simulink subsystem "startOLAE2"  (R2021a)
settings: Solver=VariableStepAuto  StartTime=0.0  StopTime=10.0  RelTol=1e-3
libraries: aerolibutil x3
settings Model: Creator=noraw  LastModifiedBy=noraw

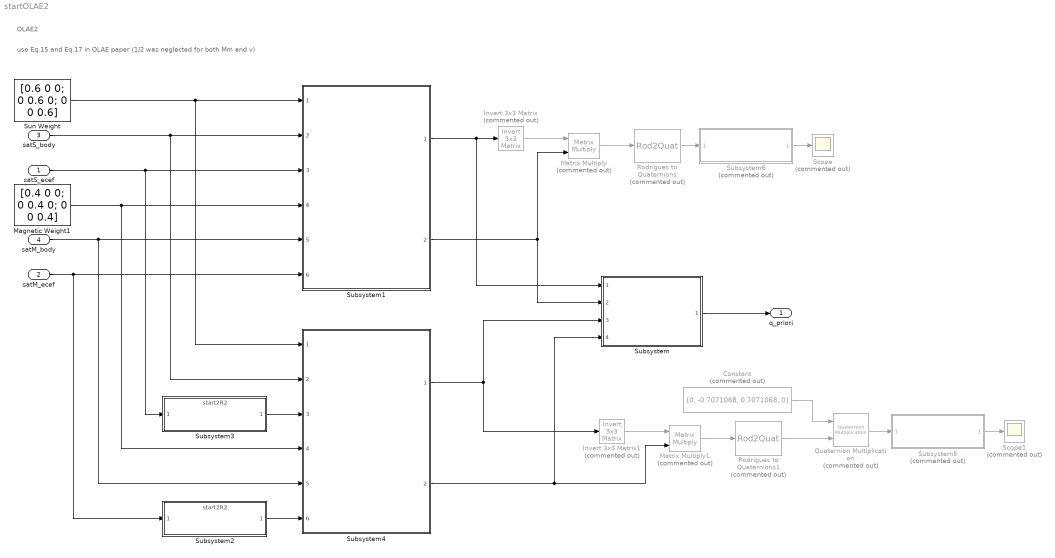
== system startOLAE2 ==
  note: OLAE2
  note: use Eq.15 and Eq.17 in OLAE paper (1/2 was neglected for both Mm and v)
  satS_ecef : Inport  PortDimensions=3
  satM_ecef : Inport  Port=2  PortDimensions=3
  satS_body : Inport  Port=3  PortDimensions=3
  satM_body : Inport  Port=4  PortDimensions=3
  Constant : Constant  Commented=on  Value=[0, -0.7071068, 0.7071068, 0]
  Invert 3x3 Matrix : aerolibutil/Invert  3x3 Matrix  Commented=on
  Invert 3x3 Matrix1 : aerolibutil/Invert  3x3 Matrix  Commented=on
  Magnetic Weight1 : Constant  Value=[0.4 0 0; 0 0.4 0; 0 0 0.4]
  Matrix Multiply : Product  Commented=on  Multiplication=Matrix(*)
  Matrix Multiply1 : Product  Commented=on  Multiplication=Matrix(*)
  Quaternion Multiplication : aerolibutil/Quaternion Multiplication  Commented=on
  Rodrigues to Quaternions : Rod2Quat  Commented=on
  Rodrigues to Quaternions1 : Rod2Quat  Commented=on
  Scope : Scope  Commented=on
  Scope1 : Scope  Commented=on
  Subsystem : Subsystem  ReferencedSubsystem=startOLAESolSelector
  Subsystem1 : Subsystem  ReferencedSubsystem=startOLAECore
  Subsystem2 : ModelReference  ModelNameDialog=start2R2  SimulationMode=Normal  ModelReferenceVersion=3.24
  Subsystem3 : ModelReference  ModelNameDialog=start2R2  SimulationMode=Normal  ModelReferenceVersion=3.24
  Subsystem4 : Subsystem  ReferencedSubsystem=startOLAECore
  Subsystem5 : Subsystem  Commented=on  ReferencedSubsystem=startQuaternionFlipper
  Subsystem6 : Subsystem  Commented=on  ReferencedSubsystem=startQuaternionFlipper
  Sun Weight : Constant  Value=[0.6 0 0; 0 0.6 0; 0 0 0.6]
  q_priori : Outport
  wires:
  Subsystem3/1 -> Subsystem4/3
  satM_ecef/1 -> Subsystem1/6, Subsystem2/1
  satM_body/1 -> Subsystem1/5, Subsystem4/5
  satS_ecef/1 -> Subsystem3/1, Subsystem1/3
  Magnetic Weight1/1 -> Subsystem1/4, Subsystem4/4
  satS_body/1 -> Subsystem1/2, Subsystem4/2
  Sun Weight/1 -> Subsystem1/1, Subsystem4/1
  Subsystem2/1 -> Subsystem4/6
  Subsystem1/2 -> Subsystem/2, Matrix Multiply/2
  Invert 3x3 Matrix/1 -> Matrix Multiply/1
  Subsystem1/1 -> Invert 3x3 Matrix/1, Subsystem/1
  Matrix Multiply/1 -> Rodrigues to Quaternions/1
  Matrix Multiply1/1 -> Rodrigues to Quaternions1/1
  Invert 3x3 Matrix1/1 -> Matrix Multiply1/1
  Subsystem4/1 -> Subsystem/3, Invert 3x3 Matrix1/1
  Subsystem4/2 -> Subsystem/4, Matrix Multiply1/2
  Quaternion Multiplication/1 -> Subsystem5/1
  Subsystem5/1 -> Scope1/1
  Subsystem6/1 -> Scope/1
  Rodrigues to Quaternions/1 -> Subsystem6/1
  Rodrigues to Quaternions1/1 -> Quaternion Multiplication/2
  Constant/1 -> Quaternion Multiplication/1
  Subsystem/1 -> q_priori/1
